simulink model "est_system"  (R2026a)
settings: Solver=VariableStepAuto

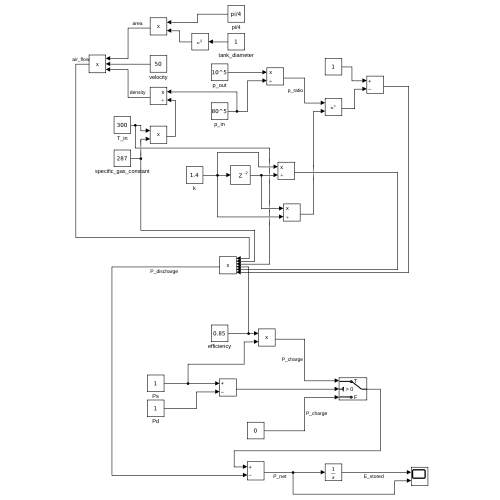
[thumbnail: Simulink's stored preview of the top-level diagram]
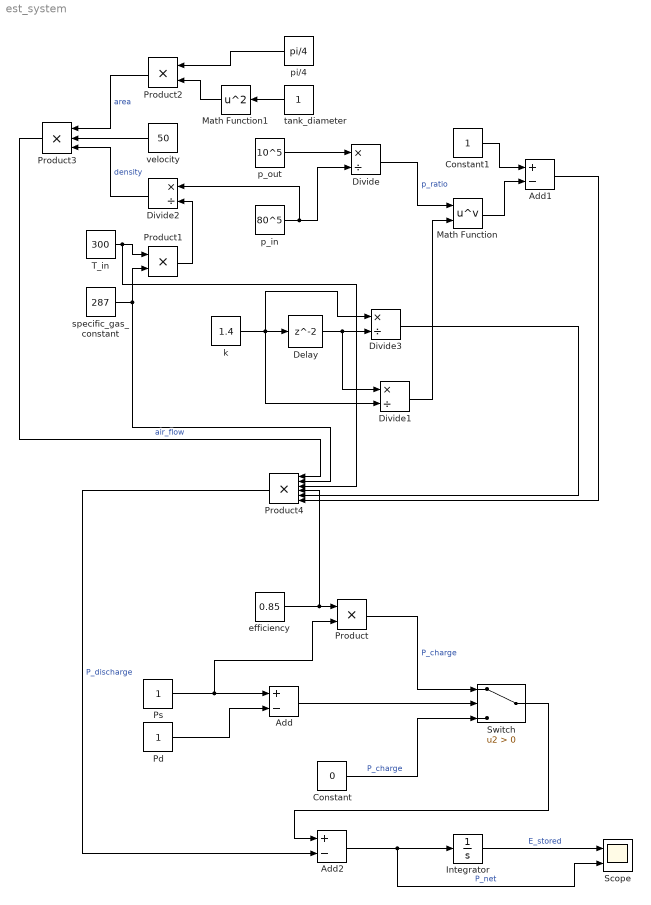
== system est_system ==
  Add : Sum  Inputs=+-
  Add1 : Sum  Inputs=+-
  Add2 : Sum  Inputs=+-
  Constant : Constant  Value=0
  Constant1 : Constant
  Delay : Delay
  Divide{,1..3} (4 alike) : Product  Inputs=*/
  Integrator : Integrator  InitialCondition=1
  Math Function : Math  Operator=pow
  Math Function1 : Math  Operator=square
  Pd : Constant
  Product : Product
  Product1 : Product
  Product2 : Product
  Product3 : Product  Inputs=3
  Product4 : Product  Inputs=6
  Ps : Constant
  Scope : Scope  NumInputPorts=2
      settings: ActiveDisplayYMinimum=0.9  ActiveDisplayYMaximum=1.1
  Switch : Switch  Criteria=u2 > Threshold  SaturateOnIntegerOverflow=off  InputSameDT=off
  T_in : Constant  Value=300
  efficiency : Constant  Value=0.85
  k : Constant  Value=1.4
  p_in : Constant  Value=80^5
  p_out : Constant  Value=10^5
  pi/4 : Constant  Value=pi/4
  specific_gas_constant : Constant  Value=287
  tank_diameter : Constant
  velocity : Constant  Value=50
  wires:
  Ps/1 -> Product/2, Add/1
  Pd/1 -> Add/2
  Add/1 -> Switch/2
  efficiency/1 -> Product4/4, Product/1
  Product/1 -> Switch/1  "P_charge"
  Constant/1 -> Switch/3  "P_charge"
  p_out/1 -> Divide/1
  p_in/1 -> Divide2/1, Divide/2
  Divide/1 -> Math Function/1  "p_ratio"
  k/1 -> Divide3/1, Divide1/2, Delay/1
  Delay/1 -> Divide3/2, Divide1/1
  Divide1/1 -> Math Function/2
  Constant1/1 -> Add1/1
  Math Function/1 -> Add1/2
  Product1/1 -> Divide2/2
  specific_gas_constant/1 -> Product4/2, Product1/2
  T_in/1 -> Product4/3, Product1/1
  Divide2/1 -> Product3/3  "density"
  tank_diameter/1 -> Math Function1/1
  pi/4/1 -> Product2/1
  Math Function1/1 -> Product2/2
  velocity/1 -> Product3/2
  Product2/1 -> Product3/1  "area"
  Product3/1 -> Product4/1  "air_flow"
  Add1/1 -> Product4/6
  Divide3/1 -> Product4/5
  Product4/1 -> Add2/2  "P_discharge"
  Switch/1 -> Add2/1
  Add2/1 -> Scope/2, Integrator/1  "P_net"
  Integrator/1 -> Scope/1  "E_stored"
